simulink model "Pure_Pursuit_with_PI"  (R2021b)
settings: Solver=VariableStepAuto  StartTime=0.0  StopTime=112  MaxStep=0.01  RelTol=1e-3
InitFcn:
  | clear all;
  | 
  | 
  | %Path in global coordinate reference frame - X and Y
  | 
  | xRef=[
  | 57.222
  | 52.707
  | 48.874
  | 44.359
  | 39.930
  | 35.160
  | 31.071
  | 16.591
  | 7.391
  | -2.575
  | -9.901
  | -13.563
  | -16.289
  | -17.567
  | -15.437
  | -8.538
  | -2.745
  | 1.002
  | 6.624
  | 10.628
  | 15.654
  | 20.935
  | 24.853
  | 28.260
  | 31.327
  | 33.797
  | 35.841
  | 36.182
  | 35.671
  | 34.478
  | 32.008
  | 29.964
  | 28.005
  | 26.301
  | 25.109
  | 24.001
  | 23.149
  | 22.383
  | 21.957
  | 21.531
  | 21.190
  | 20.850
  | 20.594
  | 21.105
  | 21.531
  | 21.701
  | 21.701
  | 21.531
  | 21.361
  | 21.446
  | 22.042
  | 23.831
  | 25.875
  | 28.771
  | ... (+154 lines)
libraries: autolibutils x4, autolibshared x2, sim3dlib x2, vehdynlibviscommon x1, slpidlib x1, simulink x1, vdynlib x1, vehdynlibsteering x1, eeGeneralControl x1, dspvision x1
(part 3 of 3)

== matlab function Pure_Pursuit_with_PI/MATLAB Function ==
  data: xRef input; yRef input; x_actual input; y_actual input; pose input; velocity input; lookahead_gain input; wheelbase input; Steering_Angle output; Steering_ratio input
function Steering_Angle    = compute(xRef, yRef, x_actual, y_actual, pose,velocity, lookahead_gain, wheelbase, Steering_ratio)

lookahead=lookahead_gain*velocity;

x_shifted=xRef-x_actual;
y_shifted=yRef-y_actual;

deg=360-((180/3.14)*pose);
matrix=[cosd(deg) -sind(deg);
        sind(deg) cosd(deg)];
K=cat(2,x_shifted,y_shifted);
K=K';
transformed=matrix*K;
x_path=transformed(1,:)-1.465;
y_path=transformed(2,:);

distance_nearest = ((x_path.^2) +(y_path.^2)).^(0.5);
[~, index_nearest] = min(distance_nearest);

distance = sqrt(x_path(index_nearest:end).^2 + y_path(index_nearest:end).^2); %finds chord length to each point
difference = distance - lookahead; %finds difference of chord lengths to lookahead
[~, index] = min(abs(difference)); %finds index and value of minimum difference
x_target = x_path(index+index_nearest); % finds X axis target value based on closest point to look ahead
y_target = y_path(index+index_nearest); % finds y axis target value based on closest point to look ahead

%calculating the curvature once again from final decided point of interest
distance_final = sqrt((y_target^2) + (x_target^2));
curvature_final = 2*y_target/((distance_final)^2);

RWA = wheelbase*curvature_final; %road wheel angle in radians
Steering_Angle=RWA*Steering_ratio;
end

== matlab function Pure_Pursuit_with_PI/Path_smoothing_function ==
  data: u1 input; xRef output; u2 input; yRef output
function [xRef,yRef] = fcn(u1,u2)

yawRef=zeros(size(u1));
directionRef=ones(size(u1));
refPoses=[u1 u2 yawRef];
refDirections=[directionRef];
numSmoothPoses=2000;
[poses,~] = smoothPathSpline(refPoses,refDirections,numSmoothPoses);

xRef=poses(:,1);
yRef=poses(:,2);



end
